simulink model "d7_cellVHT"  (R2017b)
settings: Solver=FixedStepDiscrete  StartTime=0.0  StopTime=5/30  RelTol=1e-3
PreLoadFcn:
  | if ~exist('frame10s.png')
  | createImage
  | end
PostLoadFcn:
  | R = 528;
  | C = 432;
undefined symbols (not defined in the file or in its folder): getnhood, strel
libraries: visionsinks x3, visionhdlio x2, hdlsllib x2, simulink_need_slupdate x2, visionhdlmorphops x2, visiongeotforms x1, visionsources x1, dspvision x1
settings Model: DataTypeOverride=Off  SimulationMode=accelerator  Creator=kotsuka  LastModifiedBy=kotsuka
settings DataIOCC: SaveOutput=off  SaveTime=off
settings OptimizationCC: BlockReduction=off  ConditionallyExecuteInputs=off  DefaultParameterBehavior=Inlined
settings DebuggingCC: AlgebraicLoopMsg=error  SingleTaskRateTransMsg=error  StrictBusMsg=ErrorOnBusTreatedAsVector
settings HardwareCC: ProdBitPerPointer=32  ProdBitPerSizeT=32  ProdBitPerPtrDiffT=32  ProdLargestAtomicFloat=None  ProdIntDivRoundTo=Undefined  ProdEndianess=Unspecified  ProdWordSize=32  ProdHWDeviceType=ASIC/FPGA->ASIC/FPGA  ProdEqTarget=off
settings CodeAppCC: StateflowObjectComments=on

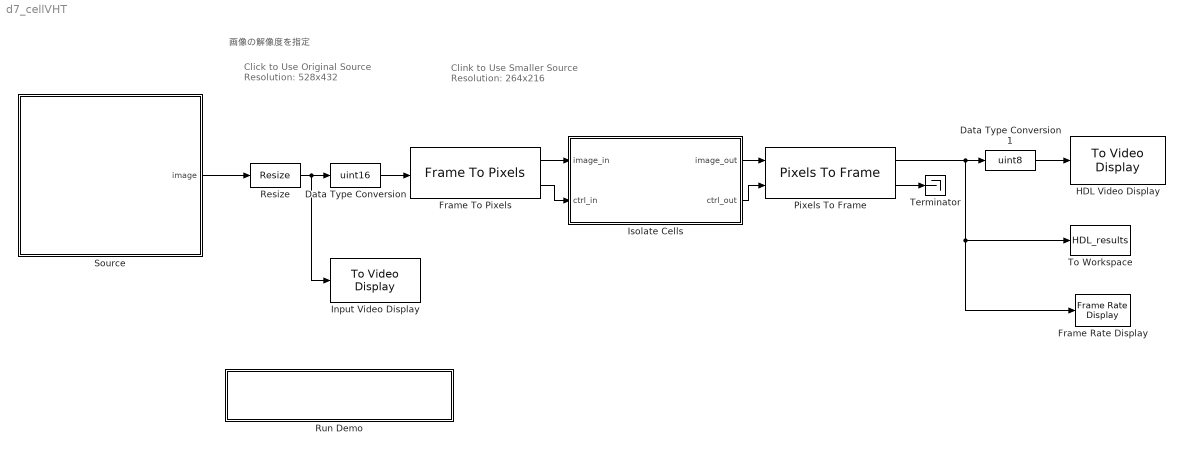
== system d7_cellVHT ==
  note: 画像の解像度を指定
  note: Click to Use Original Source
      |
      | Resolution: 528x432
  note: Clink to Use Smaller Source
      |
      | Resolution: 264x216
  Data Type Conversion : DataTypeConversion  OutDataTypeStr=uint16
  Data Type Conversion1 : DataTypeConversion  OutDataTypeStr=uint8  SaturateOnIntegerOverflow=on
  Frame Rate Display : visionsinks/Frame Rate Display  UpdateRate=2
      settings: SourceProductName=Computer Vision System Toolbox  SourceProductBaseCode=VP
  Frame To Pixels : visionhdlio/Frame To Pixels  NumComponents=1  VideoFormat=Custom  ActivePixelsPerLine=R  ActiveVideoLines=C  TotalPixelsPerLine=R+20  TotalVideoLines=C+20  StartingActiveLine=11  FrontPorch=10  SampleTime=0
      settings: SourceProductName=Vision HDL Toolbox  SourceProductBaseCode=VT
  HDL Video Display : visionsinks/To Video Display  windowSizeMode=Normal  openAtMdlStart=on  fullScreen=off  videoWindowX=1985  videoWindowY=566  saveWindowSize=off  videoWindowWidth=540  videoWindowHeight=493  inputColorFormat=RGB  inputType=Obsolete  imagePorts=One multidimensional signal  OutputDevice=On-screen video monitor  dataOrg=Column-major  isWindowOpen=off
      settings: SourceProductName=Computer Vision System Toolbox
  Input Video Display : visionsinks/To Video Display  windowSizeMode=Normal  openAtMdlStart=on  fullScreen=off  videoWindowX=1985  videoWindowY=148  saveWindowSize=off  videoWindowWidth=528  videoWindowHeight=486  inputColorFormat=RGB  inputType=Obsolete  imagePorts=One multidimensional signal  OutputDevice=On-screen video monitor  dataOrg=Column-major  isWindowOpen=off
      settings: SourceProductName=Computer Vision System Toolbox
  Isolate Cells : Subsystem  TreatAsAtomicUnit=on
  Pixels To Frame : visionhdlio/Pixels To Frame  NumComponents=1  VideoFormat=Custom  ActivePixelsPerLine=R  ActiveVideoLines=C  TotalPixelsPerLine=R+20  TotalVideoLines=C+20
      settings: SourceProductName=Vision HDL Toolbox  SourceProductBaseCode=VT
  Resize : visiongeotforms/Resize  specify=Number of output rows and columns  rfactor=[200 150]  outCols=25  outRows=25  outRowsCols=[C R]  interp_method=Bilinear  antialias=on  useROI=off  roiFlag=off  prodOutputMode=Binary point scaling  prodOutputWordLength=32  prodOutputFracLength=10  roundingMode=Nearest  overflowMode=on
      settings: SourceProductName=Computer Vision System Toolbox  SourceProductBaseCode=VP
  Run Demo : Subsystem
      settings: OpenFcn=hdladvisor([bdroot, '/Isolate Cells'])
      mask Display: disp('Launch HDL Workflow Advisor')
  Source : Subsystem
      mask Display: image(repmat(imread('frame10s.png'), [1 1 3]))
  Terminator : Terminator
  To Workspace : ToWorkspace  VariableName=HDL_results  SampleTime=-1
  wires:
  Pixels To Frame/1 -> Data Type Conversion1/1, To Workspace/1, Frame Rate Display/1
  Data Type Conversion1/1 -> HDL Video Display/1
  Pixels To Frame/2 -> Terminator/1
  Frame To Pixels/1 -> Isolate Cells/1(image_in)
  Isolate Cells/2(ctrl_out) -> Pixels To Frame/2
  Isolate Cells/1(image_out) -> Pixels To Frame/1
  Frame To Pixels/2 -> Isolate Cells/2(ctrl_in)
  Data Type Conversion/1 -> Frame To Pixels/1
  Source/1(image) -> Resize/1
  Resize/1 -> Input Video Display/1, Data Type Conversion/1

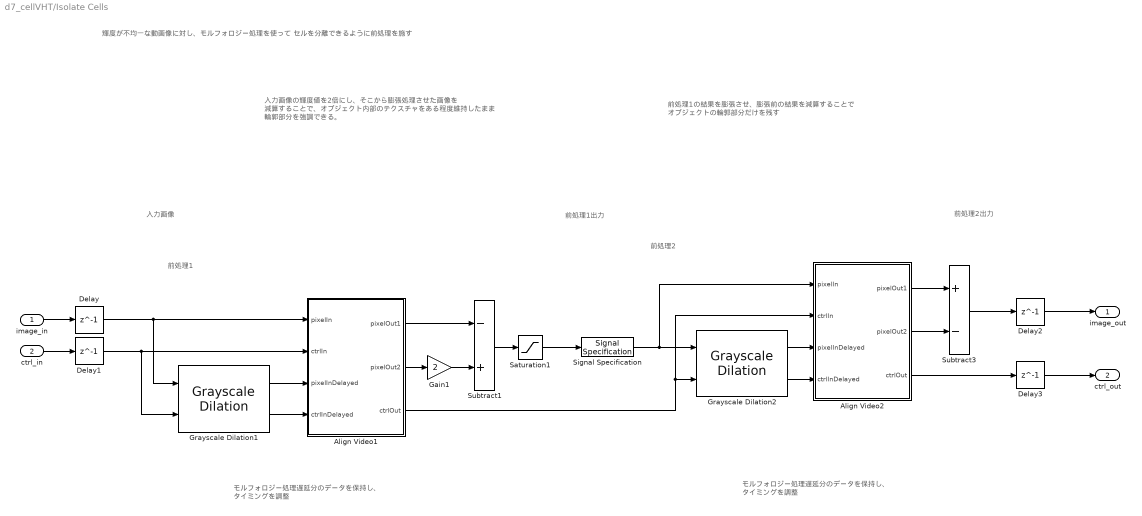
== system d7_cellVHT/Isolate Cells ==
  note: 入力画像の輝度値を2倍にし、そこから膨張処理させた画像を
      | 減算することで、オブジェクト内部のテクスチャをある程度維持したまま
      | 輪郭部分を強調できる。
  note: 前処理2出力
  note: 前処理1出力
  note: 入力画像
  note: モルフォロジー処理遅延分のデータを保持し、
      | タイミングを調整
  note: 輝度が不均一な動画像に対し、モルフォロジー処理を使って
      | セルを分離できるように前処理を施す
  note: 前処理2
  note: 前処理1
  note: モルフォロジー処理遅延分のデータを保持し、
      | タイミングを調整
  note: 前処理1の結果を膨張させ、膨張前の結果を減算することで
      | オブジェクトの輪郭部分だけを残す
  image_in : Inport
  ctrl_in : Inport  Port=2
  Align Video1 : Subsystem
  Align Video2 : Subsystem
  Delay{,1..3} (4 alike) : Delay  DelayLength=1  InitialCondition=0
  Gain1 : Gain  Gain=2  OutDataTypeStr=fixdt(0,17,0)
  Grayscale Dilation1 : visionhdlmorphops/Grayscale Dilation  Neighborhood=getnhood(strel('square',7))  LineBufferSize=2048  SimulateUsing=Code generation
      settings: SourceProductName=Vision HDL Toolbox  SourceProductBaseCode=VT
  Grayscale Dilation2 : visionhdlmorphops/Grayscale Dilation  Neighborhood=getnhood(strel('square',7))  LineBufferSize=2048  SimulateUsing=Code generation
      settings: SourceProductName=Vision HDL Toolbox  SourceProductBaseCode=VT
  Saturation1 : Saturate  UpperLimit=65535  LowerLimit=0
  Signal Specification : SignalSpecification  Dimensions=[1 1]
  Subtract1 : Sum  Inputs=-+  OutDataTypeStr=uint16  SaturateOnIntegerOverflow=on
  Subtract3 : Sum  Inputs=+-  SaturateOnIntegerOverflow=on  OutDataTypeStr=Inherit: Same as first input
  image_out : Outport
  ctrl_out : Outport  Port=2
  wires:
  Grayscale Dilation1/1 -> Align Video1/3(pixelInDelayed)
  Grayscale Dilation1/2 -> Align Video1/4(ctrlInDelayed)
  Align Video1/2(pixelOut2) -> Gain1/1
  image_in/1 -> Delay/1
  ctrl_in/1 -> Delay1/1
  Gain1/1 -> Subtract1/2
  Align Video1/1(pixelOut1) -> Subtract1/1
  Subtract1/1 -> Saturation1/1
  Saturation1/1 -> Signal Specification/1
  Align Video1/3(ctrlOut) -> Grayscale Dilation2/2, Align Video2/2(ctrlIn)
  Grayscale Dilation2/1 -> Align Video2/3(pixelInDelayed)
  Grayscale Dilation2/2 -> Align Video2/4(ctrlInDelayed)
  Align Video2/2(pixelOut2) -> Subtract3/2
  Align Video2/1(pixelOut1) -> Subtract3/1
  Subtract3/1 -> Delay2/1
  Align Video2/3(ctrlOut) -> Delay3/1
  Signal Specification/1 -> Grayscale Dilation2/1, Align Video2/1(pixelIn)
  Delay/1 -> Grayscale Dilation1/1, Align Video1/1(pixelIn)
  Delay1/1 -> Grayscale Dilation1/2, Align Video1/2(ctrlIn)
  Delay2/1 -> image_out/1
  Delay3/1 -> ctrl_out/1

== system d7_cellVHT/Run Demo ==

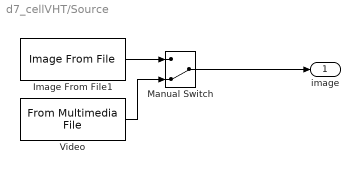
== system d7_cellVHT/Source ==
  Image From File1 : visionsources/Image From File  Tag=vipblks_nd  FileName=frame10.png  imagePorts=One multidimensional signal  Ts=1/30  ImageDataType=Inherit from input image  Signed=on  WordLength=16  sdImageDataType=uint(8)  FractionLengthMode=User-defined  FractionLength=15  OutPortLabels=R|G|B
      settings: SourceProductName=Computer Vision System Toolbox
  Manual Switch : ManualSwitch  CurrentSetting=0
  Video : dspvision/From Multimedia File  inputFilename=ecolicells.avi  loop=on  numPlays=inf  outputStreams=Video only  videoDataType=uint8  audioDataType=int16  inheritSampleTime=off  userDefinedSampleTime=1/30  noAudioOutput=off  isIntensityVideo=off  fourcc=Intensity  colorVideoFormat=Separate color signals  outputEOF=off  dataOrg=Column-major  audioFrameSize=1024  computeAudioFrameSize=off  outSamplingMode=Frame based
      settings: SourceProductBaseCode=VP
  image : Outport
  wires:
  Manual Switch/1 -> image/1
  Image From File1/1 -> Manual Switch/1
  Video/1 -> Manual Switch/2

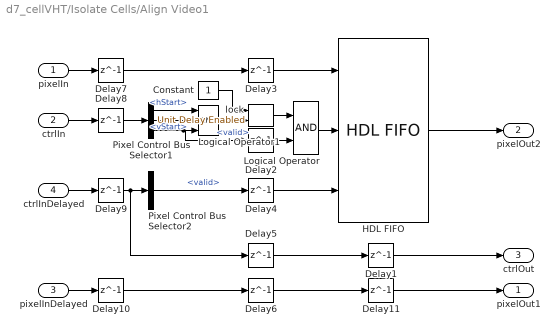
== system d7_cellVHT/Isolate Cells/Align Video1 ==
  pixelIn : Inport
  ctrlIn : Inport  Port=2
  pixelInDelayed : Inport  Port=3
  ctrlInDelayed : Inport  Port=4
  Constant : Constant  OutDataTypeStr=boolean  SampleTime=-1
  Delay{1..11} (11 alike) : Delay  DelayLength=1  InitialCondition=0
  HDL FIFO : hdlsllib/HDL RAMs/HDL FIFO  fifo_size=2048  ratio=1  push_msg=Warning  pop_msg=Warning  show_empty=off  show_full=off  show_num=off
      settings: SourceProductName=HDL Coder  SourceProductBaseCode=HD
  Logical Operator : Logic  AllPortsSameDT=off  OutDataTypeStr=boolean
  Logical Operator1 : Logic  Inputs=3  AllPortsSameDT=off  OutDataTypeStr=boolean
  Pixel Control Bus Selector1 : BusSelector  OutputSignals=hStart,vStart,valid
  Pixel Control Bus Selector2 : BusSelector  OutputSignals=valid
  lock : simulink_need_slupdate/Unit Delay Enabled  vinit=false  tsamp=-1
      settings: SourceProductName=Simulink  SourceProductBaseCode=SL
  pixelOut1 : Outport
  pixelOut2 : Outport  Port=2
  ctrlOut : Outport  Port=3
  wires:
  pixelInDelayed/1 -> Delay10/1
  HDL FIFO/1 -> pixelOut2/1
  ctrlInDelayed/1 -> Delay9/1
  ctrlIn/1 -> Delay8/1
  pixelIn/1 -> Delay7/1
  Delay6/1 -> Delay11/1
  Delay5/1 -> Delay1/1
  Delay4/1 -> HDL FIFO/3
  Delay3/1 -> HDL FIFO/1
  Pixel Control Bus Selector1/3 -> Delay2/1, Logical Operator1/3  "<valid>"
  Delay2/1 -> Logical Operator/2
  Constant/1 -> lock/1
  lock/1 -> Logical Operator/1
  Logical Operator/1 -> HDL FIFO/2
  Pixel Control Bus Selector2/1 -> Delay4/1  "<valid>"
  Delay7/1 -> Delay3/1
  Delay10/1 -> Delay6/1
  Delay8/1 -> Pixel Control Bus Selector1/1
  Delay9/1 -> Pixel Control Bus Selector2/1, Delay5/1
  Logical Operator1/1 -> lock/2
  Pixel Control Bus Selector1/2 -> Logical Operator1/2  "<vStart>"
  Pixel Control Bus Selector1/1 -> Logical Operator1/1  "<hStart>"
  Delay1/1 -> ctrlOut/1
  Delay11/1 -> pixelOut1/1

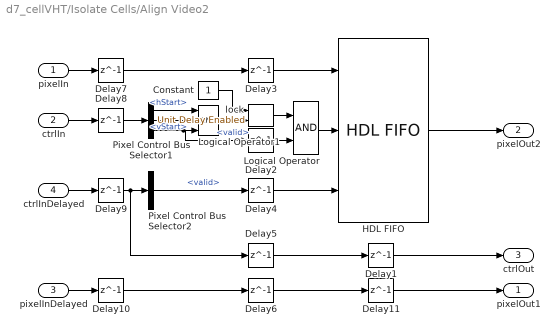
== system d7_cellVHT/Isolate Cells/Align Video2 ==
  pixelIn : Inport
  ctrlIn : Inport  Port=2
  pixelInDelayed : Inport  Port=3
  ctrlInDelayed : Inport  Port=4
  Constant : Constant  OutDataTypeStr=boolean  SampleTime=-1
  Delay{1..11} (11 alike) : Delay  DelayLength=1  InitialCondition=0
  HDL FIFO : hdlsllib/HDL RAMs/HDL FIFO  fifo_size=2048  ratio=1  push_msg=Warning  pop_msg=Warning  show_empty=off  show_full=off  show_num=off
      settings: SourceProductName=HDL Coder  SourceProductBaseCode=HD
  Logical Operator : Logic  AllPortsSameDT=off  OutDataTypeStr=boolean
  Logical Operator1 : Logic  Inputs=3  AllPortsSameDT=off  OutDataTypeStr=boolean
  Pixel Control Bus Selector1 : BusSelector  OutputSignals=hStart,vStart,valid
  Pixel Control Bus Selector2 : BusSelector  OutputSignals=valid
  lock : simulink_need_slupdate/Unit Delay Enabled  vinit=false  tsamp=-1
      settings: SourceProductName=Simulink  SourceProductBaseCode=SL
  pixelOut1 : Outport
  pixelOut2 : Outport  Port=2
  ctrlOut : Outport  Port=3
  wires:
  Delay11/1 -> pixelOut1/1
  Delay1/1 -> ctrlOut/1
  Pixel Control Bus Selector1/1 -> Logical Operator1/1  "<hStart>"
  Pixel Control Bus Selector1/2 -> Logical Operator1/2  "<vStart>"
  Logical Operator1/1 -> lock/2
  Delay9/1 -> Delay5/1, Pixel Control Bus Selector2/1
  Delay8/1 -> Pixel Control Bus Selector1/1
  Delay10/1 -> Delay6/1
  Delay7/1 -> Delay3/1
  Pixel Control Bus Selector2/1 -> Delay4/1  "<valid>"
  Logical Operator/1 -> HDL FIFO/2
  lock/1 -> Logical Operator/1
  Constant/1 -> lock/1
  Delay2/1 -> Logical Operator/2
  Pixel Control Bus Selector1/3 -> Logical Operator1/3, Delay2/1  "<valid>"
  Delay3/1 -> HDL FIFO/1
  Delay4/1 -> HDL FIFO/3
  Delay5/1 -> Delay1/1
  Delay6/1 -> Delay11/1
  pixelIn/1 -> Delay7/1
  ctrlIn/1 -> Delay8/1
  ctrlInDelayed/1 -> Delay9/1
  HDL FIFO/1 -> pixelOut2/1
  pixelInDelayed/1 -> Delay10/1
